simulink model "untitled"  (R2022b)
settings: Solver=VariableStepAuto  StartTime=0.0  StopTime=10.0  RelTol=1e-3
settings Model: Creator=Nhan  LastModifiedBy=Nhan

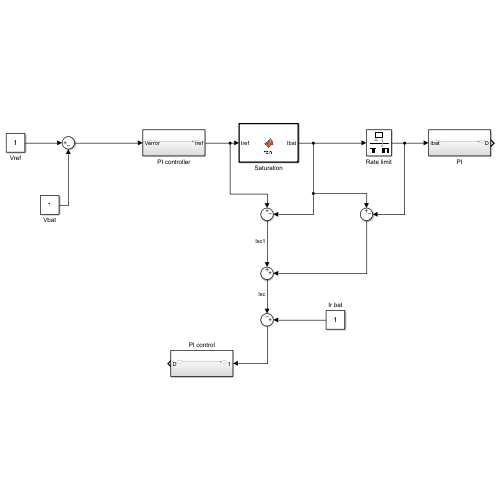
[thumbnail: Simulink's stored preview of the top-level diagram]
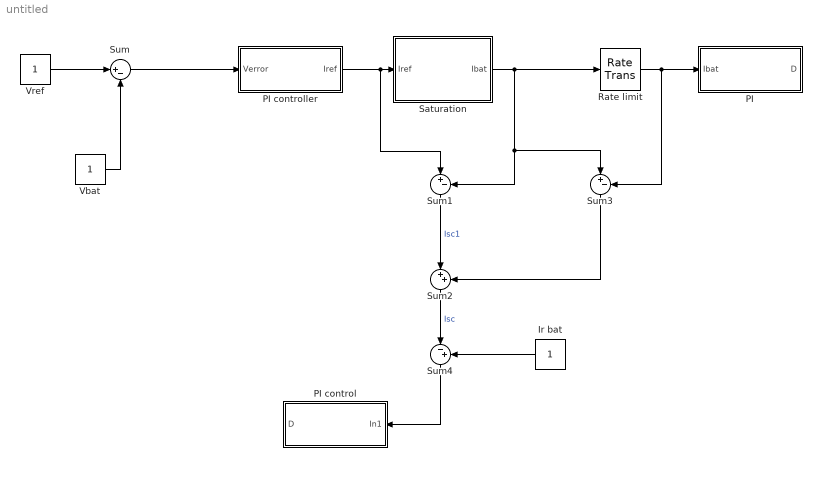
== system untitled ==
  Ir bat : Constant
  PI : Subsystem
  PI control : Subsystem
  PI controller : Subsystem
  Rate limit : RateTransition  OutPortSampleTime=1e-3
  Saturation : MATLAB Function  TreatAsAtomicUnit=on
  Sum : Sum  Inputs=|+-
  Sum1 : Sum  Inputs=|+-
  Sum2 : Sum  Inputs=|++
  Sum3 : Sum  Inputs=|+-
  Sum4 : Sum  Inputs=|-+
  Vbat : Constant
  Vref : Constant
  wires:
  Vref/1 -> Sum/1
  Vbat/1 -> Sum/2
  Sum/1 -> PI controller/1(Verror)
  PI controller/1(Iref) -> Sum1/1, Saturation/1(Iref)
  Saturation/1(Ibat) -> Rate limit/1, Sum1/2, Sum3/1
  Rate limit/1 -> Sum3/2, PI/1(Ibat)
  Sum1/1 -> Sum2/1  "Isc1"
  Sum3/1 -> Sum2/2
  Sum2/1 -> Sum4/1  "Isc"
  Ir bat/1 -> Sum4/2
  Sum4/1 -> PI control/1(In1)

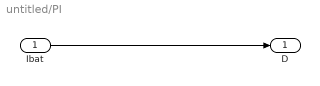
== system untitled/PI ==
  Ibat : Inport
  D : Outport
  wires:
  Ibat/1 -> D/1

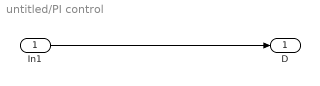
== system untitled/PI control ==
  In1 : Inport
  D : Outport
  wires:
  In1/1 -> D/1

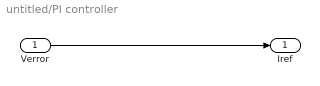
== system untitled/PI controller ==
  Verror : Inport
  Iref : Outport
  wires:
  Verror/1 -> Iref/1

== matlab function untitled/Saturation ==
  data: Iref input; Ibat output
function Ibat = fcn(Iref)
    if Iref < 4
        Ibat = Iref;
    else
        Ibat = 4;
    end
end
